simulink model "modelo_p1_2014"  (R2025a)
settings: Solver=VariableStepAuto  StartTime=0.0  StopTime=10.0  RelTol=1e-3
libraries: simulink x3
settings Model: Creator=joaof  LastModifiedBy=joaof

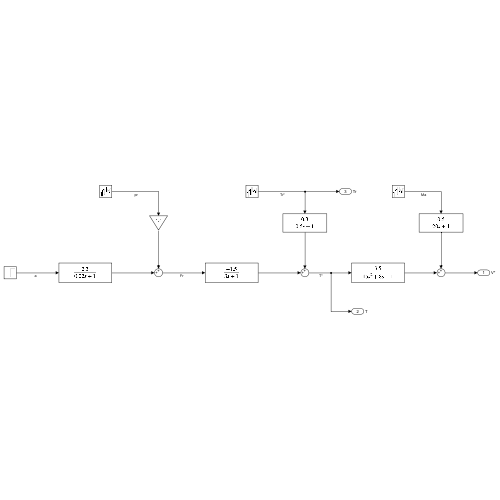
[thumbnail: Simulink's stored preview of the top-level diagram]
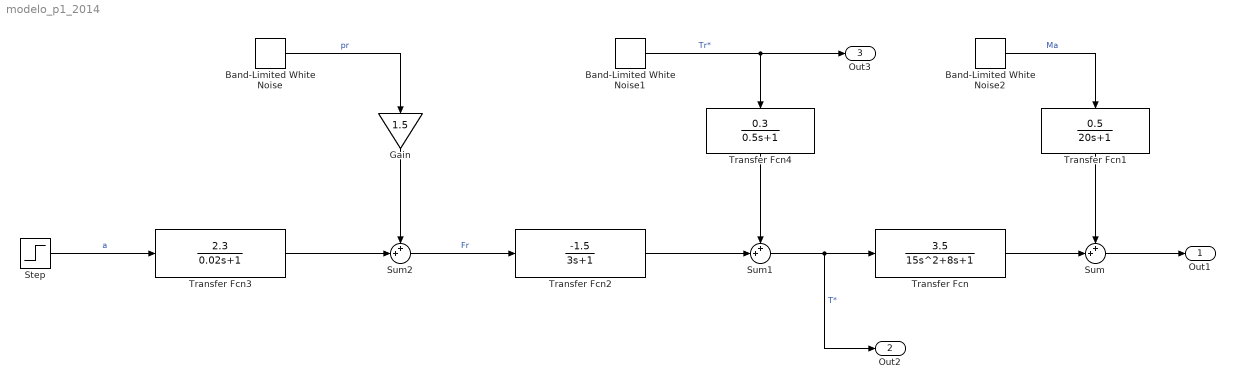
== system modelo_p1_2014 ==
  Band-Limited White Noise : simulink/Sources/Band-Limited White Noise  Cov=[0.1]  Ts=0.1  seed=[23341]
  Band-Limited White Noise1 : simulink/Sources/Band-Limited White Noise  Cov=[0.1]  Ts=0.1  seed=[23341]
  Band-Limited White Noise2 : simulink/Sources/Band-Limited White Noise  Cov=[0.1]  Ts=0.1  seed=[23341]
  Gain : Gain  Gain=1.5
  Step : Step  SampleTime=0
  Sum : Sum  Inputs=++|
  Sum1 : Sum  Inputs=++|
  Sum2 : Sum  Inputs=++|
  Transfer Fcn : TransferFcn  Numerator=[3.5]  Denominator=[15 8 1]
  Transfer Fcn1 : TransferFcn  Numerator=[0.5]  Denominator=[20 1]
  Transfer Fcn2 : TransferFcn  Numerator=[-1.5]  Denominator=[3 1]
  Transfer Fcn3 : TransferFcn  Numerator=[2.3]  Denominator=[0.02 1]
  Transfer Fcn4 : TransferFcn  Numerator=[0.3]  Denominator=[0.5 1]
  Out1 : Outport  SignalName=V*
  Out2 : Outport  Port=2  SignalName=T
  Out3 : Outport  Port=3  SignalName=Tr
  wires:
  Transfer Fcn1/1 -> Sum/1
  Transfer Fcn/1 -> Sum/2
  Transfer Fcn2/1 -> Sum1/2
  Sum1/1 -> Out2/1, Transfer Fcn/1  "T*"
  Transfer Fcn4/1 -> Sum1/1
  Transfer Fcn3/1 -> Sum2/2
  Sum2/1 -> Transfer Fcn2/1  "Fr"
  Gain/1 -> Sum2/1
  Band-Limited White Noise/1 -> Gain/1  "pr"
  Step/1 -> Transfer Fcn3/1  "a"
  Band-Limited White Noise1/1 -> Out3/1, Transfer Fcn4/1  "Tr*"
  Band-Limited White Noise2/1 -> Transfer Fcn1/1  "Ma"
  Sum/1 -> Out1/1
